simulink model "V7Callback"  (R2020b)
settings: Solver=FixedStepAuto  StartTime=0.0  StopTime=20.0  FixedStep=0.1  MaxStep=0.1  MinStep=0.1  RelTol=1e-3  EnableMultiTasking=on
PreLoadFcn:
  | V7SetParam
values from neighbouring files (symbols this model uses):
  c1 = c    (= 1)    [V1SetParam.m]    (also in V3VektorSetParam.m; V7Callback_2018_05_25_18_20_53_343.mat; V7SetParam.m; myData.mat)
  c2 = c    (= 1)    [V1SetParam.m]    (also in V3VektorSetParam.m; V7Callback_2018_05_25_18_20_53_343.mat; V7SetParam.m)
  c3 = c    (= 1)    [V1SetParam.m]    (also in V3VektorSetParam.m; V7Callback_2018_05_25_18_20_53_343.mat; V7SetParam.m)
  c4 = c    (= 1)    [V1SetParam.m]    (also in V3VektorSetParam.m; V7Callback_2018_05_25_18_20_53_343.mat; V7SetParam.m)
  m1 = m    (= 2)    [V1SetParam.m]    (also in V3VektorSetParam.m; V7Callback_2018_05_25_18_20_53_343.mat; V7SetParam.m; myData.mat)
  m2 = m    (= 2)    [V1SetParam.m]    (also in V3VektorSetParam.m; V7Callback_2018_05_25_18_20_53_343.mat; V7SetParam.m)
  m3 = m    (= 2)    [V1SetParam.m]    (also in V3VektorSetParam.m; V7Callback_2018_05_25_18_20_53_343.mat; V7SetParam.m)
  v1 = 0    [V7Callback_2018_05_25_18_20_53_343.mat]    (also in V7SetParam.m)
  v10 = 0    [V1SetParam.m]
  v2 = 0    [V7Callback_2018_05_25_18_20_53_343.mat]    (also in V7SetParam.m)
  v20 = 0    [V1SetParam.m]
  v3 = 0    [V7Callback_2018_05_25_18_20_53_343.mat]    (also in V7SetParam.m)
  v30 = 0    [V1SetParam.m]
  x1 = -1    [V7Callback_2018_05_25_18_20_53_343.mat]    (also in V7SetParam.m)
  x10 = -1    [V1SetParam.m]
  x2 = 0    [V7Callback_2018_05_25_18_20_53_343.mat]    (also in V7SetParam.m)
  x20 = 0    [V1SetParam.m]
  x3 = 1    [V7Callback_2018_05_25_18_20_53_343.mat]    (also in V7SetParam.m)
  x30 = 1    [V1SetParam.m]
settings Model: Creator=Reichl  LastModifiedBy=jakob
settings DataIOCC: SaveFormat=Array  SignalLoggingSaveFormat=ModelDataLogs  ReturnWorkspaceOutputs=off
settings OptimizationCC: ExpressionDepthLimit=2147483647  LifeSpan=inf
settings DebuggingCC: UnderspecifiedInitializationDetection=Classic  MergeDetectMultiDrivingBlocksExec=none  SolverPrmCheckMsg=warning  FcnCallInpInsideContextMsg=warning  AllowSymbolicDim=off  StateNameClashWarn=warning  SFUnexpectedBacktrackingDiag=warning  SFNoUnconditionalDefaultTransitionDiag=warning  SFExecutionAtInitializationDiag=none  ArithmeticOperatorsInVariantConditions=warning
settings HardwareCC: ProdBitPerPointer=32  ProdBitPerSizeT=32  ProdBitPerPtrDiffT=32  ProdLargestAtomicFloat=None  ProdIntDivRoundTo=Undefined  ProdEndianess=Unspecified  ProdWordSize=32  ProdHWDeviceType=32-bit Generic
settings ModelReferenceCC: PropagateSignalLabelsOutOfModel=off
settings SFSimCC: SimUseLocalCustomCode=off  CustomCodeUndefinedFunction=UseInterfaceOnly
settings RTWCC: RTWUseLocalCustomCode=off
settings CodeAppCC: StateflowObjectComments=on
settings GRTTargetCC: TargetLangStandard=C89/C90 (ANSI)  CombineOutputUpdateFcns=off  GRTInterface=on
settings ConfigComp: CovMetricSettings=dw  CovSaveCumulativeToWorkspaceVar=on  CovSaveSingleToWorkspaceVar=on  CovExternalEMLEnable=off  CovSFcnEnable=off

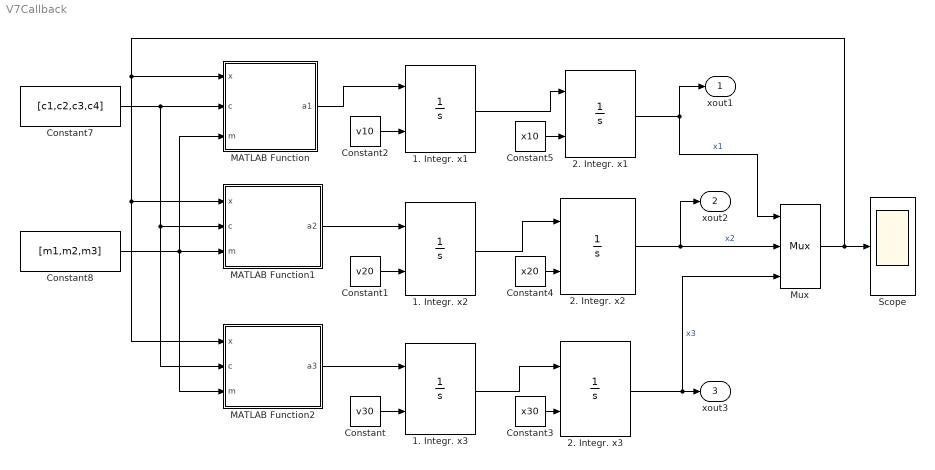
== system V7Callback ==
  1. Integr. x1 : Integrator  InitialConditionSource=external  InitialCondition=v1
  1. Integr. x2 : Integrator  InitialConditionSource=external  InitialCondition=v2
  1. Integr. x3 : Integrator  InitialConditionSource=external  InitialCondition=v3
  2. Integr. x1 : Integrator  InitialConditionSource=external  InitialCondition=x1
  2. Integr. x2 : Integrator  InitialConditionSource=external  InitialCondition=x2
  2. Integr. x3 : Integrator  InitialConditionSource=external  InitialCondition=x3
  Constant : Constant  Value=v30
  Constant1 : Constant  Value=v20
  Constant2 : Constant  Value=v10
  Constant3 : Constant  Value=x30
  Constant4 : Constant  Value=x20
  Constant5 : Constant  Value=x10
  Constant7 : Constant  Value=[c1,c2,c3,c4]
  Constant8 : Constant  Value=[m1,m2,m3]
  MATLAB Function : MATLAB Function  TreatAsAtomicUnit=on
  MATLAB Function1 : MATLAB Function  TreatAsAtomicUnit=on
  MATLAB Function2 : MATLAB Function  TreatAsAtomicUnit=on
  Mux : Mux  Inputs=3
      settings: DisplayOption=signals
  Scope : Scope
  xout1 : Outport  VectorParamsAs1DForOutWhenUnconnected=off
  xout2 : Outport  Port=2  VectorParamsAs1DForOutWhenUnconnected=off
  xout3 : Outport  Port=3  VectorParamsAs1DForOutWhenUnconnected=off
  wires:
  1. Integr. x1/1 -> 2. Integr. x1/1
  1. Integr. x2/1 -> 2. Integr. x2/1
  1. Integr. x3/1 -> 2. Integr. x3/1
  2. Integr. x2/1 -> Mux/2, xout2/1  "x2"
  2. Integr. x1/1 -> Mux/1, xout1/1  "x1"
  2. Integr. x3/1 -> Mux/3, xout3/1  "x3"
  MATLAB Function/1(a1) -> 1. Integr. x1/1
  MATLAB Function1/1(a2) -> 1. Integr. x2/1
  MATLAB Function2/1(a3) -> 1. Integr. x3/1
  Mux/1 -> Scope/1, MATLAB Function2/1(x), MATLAB Function1/1(x), MATLAB Function/1(x)
  Constant7/1 -> MATLAB Function2/2(c), MATLAB Function1/2(c), MATLAB Function/2(c)
  Constant8/1 -> MATLAB Function/3(m), MATLAB Function2/3(m), MATLAB Function1/3(m)
  Constant3/1 -> 2. Integr. x3/2
  Constant5/1 -> 2. Integr. x1/2
  Constant4/1 -> 2. Integr. x2/2
  Constant/1 -> 1. Integr. x3/2
  Constant1/1 -> 1. Integr. x2/2
  Constant2/1 -> 1. Integr. x1/2

== matlab function V7Callback/MATLAB Function1 ==
  data: x input; c input; a2 output; m input
function a2 = fcn(x, c, m)
a2 = -( c(2)*(x(2)-x(1)) + c(3)*(x(2)-x(3)) )/m(2);

== matlab function V7Callback/MATLAB Function ==
  data: x input size=[3,1]; a1 output; c input; m input
function a1 = fcn(x,c,m)
a1 = -( c(1)*x(1) + c(2)*(x(1)-x(2)) ) / m(1);

== matlab function V7Callback/MATLAB Function2 ==
  data: x input; c input; m input; a3 output
function a3 = fcn(x,c,m)
a3 = -( c(3)*(x(3)-x(2)) + c(4)*x(3) )/m(3);
